simulink model "micromodelswil"  (R2021a)
settings: Solver=FixedStepAuto  StartTime=0.0  StopTime=inf  FixedStep=0.05  RelTol=1e-3
undefined symbols (not defined in the file): Angular, Linear
libraries: robotlib x21
settings Model: Creator=refulgent  LastModifiedBy=refulgent
settings OptimizationCC: EnhancedBackFolding=on  PassReuseOutputArgsAs=Individual arguments  ZeroExternalMemoryAtStartup=off  ZeroInternalMemoryAtStartup=off  MaxStackSize=64  OptimizeBlockOrder=speed  DifferentSizesBufferReuse=on  OptimizationCustomize=off  EfficientTunableParamExpr=on
settings DebuggingCC: ParameterTunabilityLossMsg=error
settings HardwareCC: ProdBitPerPointer=32  ProdBitPerSizeT=32  ProdBitPerPtrDiffT=32  ProdLargestAtomicFloat=None  ProdIntDivRoundTo=Undefined  ProdEndianess=Unspecified  ProdWordSize=32  ProdHWDeviceType=Generic->Unspecified (assume 32-bit Generic)
settings SFSimCC: MATLABDynamicMemAlloc=off
settings RTWCC: SystemTargetFile=ert.tlc  HardwareBoard=Robot Operating System (ROS)  TLCOptions="-aInlineSetEventsForThisBaseRateFcn=TLC_FALSE -aSuppressMultiTaskScheduler=TLC_FALSE  -aRateBasedStepFcn=0"  TemplateMakefile=ert_default_tmf  Toolchain=Catkin  TargetLang=C++
settings CodeAppCC: ForceParamTrailComments=on  IgnoreCustomStorageClasses=off  OperatorAnnotations=on  SimulinkDataObjDesc=on  SFDataObjDesc=on  InsertBlockDesc=on

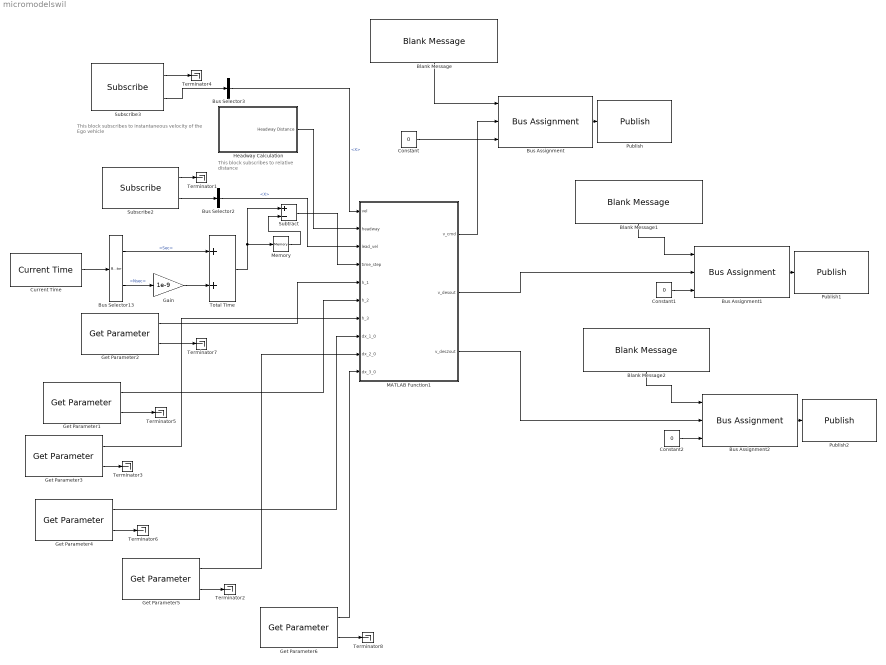
== system micromodelswil ==
  note: This block subscribes to
      | instantaneous velocity of the Ego vehicle
  note: This block subscribes
      | to relative distance
  Blank Message : robotlib/Blank Message  messageClass=Message  entityType=geometry_msgs/Twist  messageType=geometry_msgs/Twist  SampleTime=inf  legacyBusStruct=off
  Blank Message1 : robotlib/Blank Message  messageClass=Message  entityType=geometry_msgs/Twist  messageType=geometry_msgs/Twist  SampleTime=inf  legacyBusStruct=off
  Blank Message2 : robotlib/Blank Message  messageClass=Message  entityType=geometry_msgs/Twist  messageType=geometry_msgs/Twist  SampleTime=inf  legacyBusStruct=off
  Bus Assignment : BusAssignment  AssignedSignals=Linear.X,Angular.Z
  Bus Assignment1 : BusAssignment  AssignedSignals=Linear.X,Angular.Z
  Bus Assignment2 : BusAssignment  AssignedSignals=Linear.X,Angular.Z
  Bus Selector13 : BusSelector  OutputSignals=Sec,Nsec
  Bus Selector2 : BusSelector  OutputSignals=Linear.X
  Bus Selector3 : BusSelector  OutputSignals=Linear.X
  Constant : Constant  Value=0
  Constant1 : Constant  Value=0
  Constant2 : Constant  Value=0
  Current Time : robotlib/Current Time  OutputFormat=bus  SampleTime=-1  ModelName=micromodelswil
      settings: SourceProductBaseCode=RR
  Gain : Gain  Gain=1e-9
  Get Parameter1 : robotlib/Get Parameter  ParameterSource=Specify your own  ParameterName=th2  ParameterType=double  ParameterMaxArrayLength=16  ParameterInitialValue=1.2  SampleTime=-1  ShowErrorCodeOutput=on  ModelName=micromodelswil  BlockId=ParamGet_micromodelswil_55
      settings: SourceProductBaseCode=RR
  Get Parameter2 : robotlib/Get Parameter  ParameterSource=Specify your own  ParameterName=th1  ParameterType=double  ParameterMaxArrayLength=16  ParameterInitialValue=0.4  SampleTime=-1  ShowErrorCodeOutput=on  ModelName=micromodelswil  BlockId=ParamGet_micromodelswil_56
      settings: SourceProductBaseCode=RR
  Get Parameter3 : robotlib/Get Parameter  ParameterSource=Specify your own  ParameterName=th3  ParameterType=double  ParameterMaxArrayLength=16  ParameterInitialValue=1.8  SampleTime=-1  ShowErrorCodeOutput=on  ModelName=micromodelswil  BlockId=ParamGet_micromodelswil_57
      settings: SourceProductBaseCode=RR
  Get Parameter4 : robotlib/Get Parameter  ParameterSource=Specify your own  ParameterName=w1  ParameterType=double  ParameterMaxArrayLength=16  ParameterInitialValue=4.5  SampleTime=-1  ShowErrorCodeOutput=on  ModelName=micromodelswil  BlockId=ParamGet_micromodelswil_58
      settings: SourceProductBaseCode=RR
  Get Parameter5 : robotlib/Get Parameter  ParameterSource=Specify your own  ParameterName=w2  ParameterType=double  ParameterMaxArrayLength=16  ParameterInitialValue=5.25  SampleTime=-1  ShowErrorCodeOutput=on  ModelName=micromodelswil  BlockId=ParamGet_micromodelswil_73
      settings: SourceProductBaseCode=RR
  Get Parameter6 : robotlib/Get Parameter  ParameterSource=Specify your own  ParameterName=w3  ParameterType=double  ParameterMaxArrayLength=16  ParameterInitialValue=6.0  SampleTime=-1  ShowErrorCodeOutput=on  ModelName=micromodelswil  BlockId=ParamGet_micromodelswil_75
      settings: SourceProductBaseCode=RR
  Headway Calculation : Subsystem
  MATLAB Function1 : MATLAB Function  TreatAsAtomicUnit=on
  Memory : Memory
  Publish : robotlib/Publish  topicSource=Specify your own  topic=cmd_vel  messageType=geometry_msgs/Twist  legacyBusStruct=off  messageQueueLength=1
  Publish1 : robotlib/Publish  topicSource=Specify your own  topic=v_des  messageType=geometry_msgs/Twist  legacyBusStruct=off  messageQueueLength=1
  Publish2 : robotlib/Publish  topicSource=Specify your own  topic=v_des2  messageType=geometry_msgs/Twist  legacyBusStruct=off  messageQueueLength=1
  Subscribe2 : robotlib/Subscribe  topicSource=Specify your own  topic=leader_vel  messageType=geometry_msgs/Twist  SampleTime=-1  legacyBusStruct=off  messageQueueLength=1
  Subscribe3 : robotlib/Subscribe  topicSource=Specify your own  topic=vel  messageType=geometry_msgs/Twist  SampleTime=-1  legacyBusStruct=off  messageQueueLength=1
  Subtract : Sum  Inputs=+-
  Terminator{1..8} (8 alike) : Terminator
  Total Time : Sum
  wires:
  Bus Selector13/2 -> Gain/1  "<Nsec>"
  Bus Selector13/1 -> Total Time/1  "<Sec>"
  Gain/1 -> Total Time/2
  Current Time/1 -> Bus Selector13/1
  Total Time/1 -> Memory/1, Subtract/1
  Memory/1 -> Subtract/2
  Subtract/1 -> MATLAB Function1/4(time_step)
  Subscribe3/1 -> Terminator4/1
  Subscribe3/2 -> Bus Selector3/1
  Bus Selector3/1 -> MATLAB Function1/1(vel)  "<X>"
  Bus Assignment/1 -> Publish/1
  Constant/1 -> Bus Assignment/3
  MATLAB Function1/1(v_cmd) -> Bus Assignment/2
  Blank Message/1 -> Bus Assignment/1
  Subscribe2/1 -> Terminator1/1
  Bus Selector2/1 -> MATLAB Function1/3(lead_vel)  "<X>"
  Subscribe2/2 -> Bus Selector2/1
  Headway Calculation/1(Headway Distance) -> MATLAB Function1/2(headway)
  Get Parameter3/2 -> Terminator3/1
  Get Parameter1/1 -> MATLAB Function1/6(h_2)
  Get Parameter3/1 -> MATLAB Function1/7(h_3)
  Get Parameter1/2 -> Terminator5/1
  Get Parameter2/1 -> MATLAB Function1/5(h_1)
  Get Parameter4/2 -> Terminator6/1
  Get Parameter2/2 -> Terminator7/1
  Get Parameter4/1 -> MATLAB Function1/8(dx_1_0)
  Blank Message1/1 -> Bus Assignment1/1
  MATLAB Function1/2(v_desout) -> Bus Assignment1/2
  Constant1/1 -> Bus Assignment1/3
  Bus Assignment1/1 -> Publish1/1
  Bus Assignment2/1 -> Publish2/1
  Constant2/1 -> Bus Assignment2/3
  MATLAB Function1/3(v_des2out) -> Bus Assignment2/2
  Blank Message2/1 -> Bus Assignment2/1
  Get Parameter5/1 -> MATLAB Function1/9(dx_2_0)
  Get Parameter5/2 -> Terminator2/1
  Get Parameter6/2 -> Terminator8/1
  Get Parameter6/1 -> MATLAB Function1/10(dx_3_0)

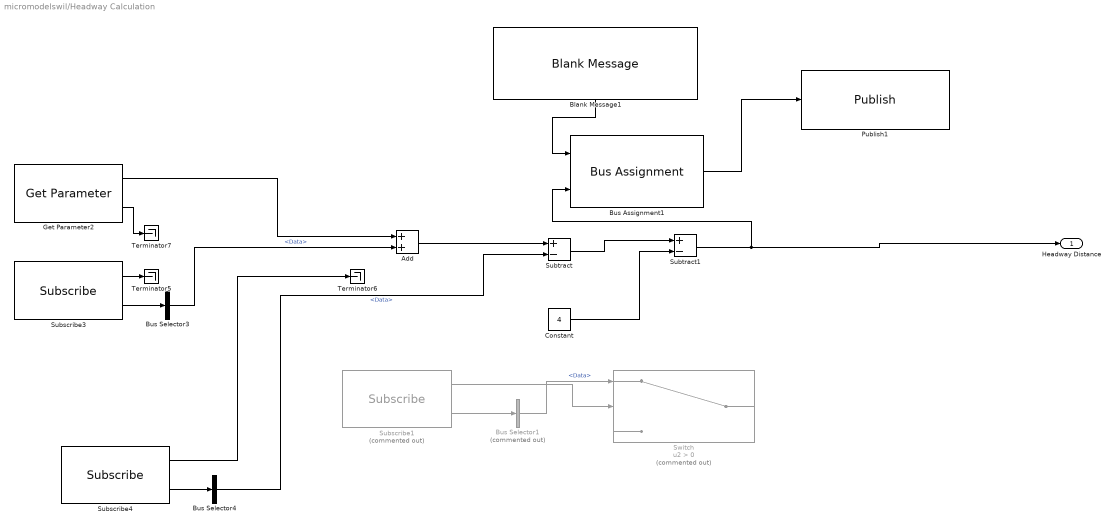
== system micromodelswil/Headway Calculation ==
  Add : Sum
  Blank Message1 : robotlib/Blank Message  messageClass=Message  entityType=std_msgs/Float64  messageType=std_msgs/Float64  SampleTime=inf  legacyBusStruct=off
  Bus Assignment1 : BusAssignment  AssignedSignals=Data
  Bus Selector1 : BusSelector  Commented=on  OutputSignals=Data
  Bus Selector3 : BusSelector  OutputSignals=Data
  Bus Selector4 : BusSelector  OutputSignals=Data
  Constant : Constant  Value=4
  Get Parameter2 : robotlib/Get Parameter  ParameterSource=Specify your own  ParameterName=init_gap  ParameterType=double  ParameterMaxArrayLength=16  ParameterInitialValue=30.0  SampleTime=-1  ShowErrorCodeOutput=on  ModelName=micromodelswil  BlockId=ParamGet_micromodelswil_39
      settings: SourceProductBaseCode=RR
  Publish1 : robotlib/Publish  topicSource=Specify your own  topic=headway_est  messageType=std_msgs/Float64  legacyBusStruct=off  messageQueueLength=1
  Subscribe1 : robotlib/Subscribe  Commented=on  topicSource=Specify your own  topic=headway  messageType=std_msgs/Float64  SampleTime=-1  legacyBusStruct=off  messageQueueLength=1
  Subscribe3 : robotlib/Subscribe  topicSource=Specify your own  topic=leader_dist_x  messageType=std_msgs/Float64  SampleTime=-1  legacyBusStruct=off  messageQueueLength=1
  Subscribe4 : robotlib/Subscribe  topicSource=Specify your own  topic=dist_x  messageType=std_msgs/Float64  SampleTime=-1  legacyBusStruct=off  messageQueueLength=1
  Subtract : Sum  Inputs=+-
  Subtract1 : Sum  Inputs=+-
  Switch : Switch  Commented=on  Criteria=u2 > Threshold
  Terminator5 : Terminator
  Terminator6 : Terminator
  Terminator7 : Terminator
  Headway Distance : Outport
  wires:
  Bus Selector3/1 -> Add/2  "<Data>"
  Subscribe1/2 -> Bus Selector1/1
  Subscribe3/2 -> Bus Selector3/1
  Subscribe4/1 -> Terminator6/1
  Bus Selector1/1 -> Switch/1  "<Data>"
  Subscribe1/1 -> Switch/2
  Bus Selector4/1 -> Subtract/2  "<Data>"
  Get Parameter2/2 -> Terminator7/1
  Subscribe4/2 -> Bus Selector4/1
  Get Parameter2/1 -> Add/1
  Subscribe3/1 -> Terminator5/1
  Add/1 -> Subtract/1
  Subtract/1 -> Subtract1/1
  Blank Message1/1 -> Bus Assignment1/1
  Bus Assignment1/1 -> Publish1/1
  Subtract1/1 -> Bus Assignment1/2, Headway Distance/1
  Constant/1 -> Subtract1/2

== matlab function micromodelswil/MATLAB Function1 ==
  data: vel input; v_cmd output; v_desout output; headway input; lead_vel input; time_step input; h_1 input; h_2 input; h_3 input; dx_1_0 input; v_des2out output; dx_2_0 input; dx_3_0 input
function [v_cmd, v_desout, v_des2out]  = Micromodel(vel, headway, lead_vel, time_step, h_1, h_2, h_3, dx_1_0, dx_2_0, dx_3_0)
%% Compute the desired acceleration by the Micromodel controller.
% This model requires memory from previous time steps to properly function.
% To achieve this, we pass the variables to be stored in memory as inputs
% to the function, and return the updated values as outputs from it. These
% parameters should be initialized as follows:
% >>> d1 = 1;
% >>> d2 = 1;
% >>> v_des2 = -1;
% >>> time_avg_target = [];
% If you would like to convert this model from an acceleration controller
% to a velocity controller, simply replace "acceleration" in the above
% function definition with "v_cmd".
% Parameters
% ----------
% vel : float
%     the speed of the ego vehicle
% headway : float
%     bumper-to-bumper gap
% lead_vel : float
%     speed of vehicle in front
% time_step : float
%     the average time (in seconds) in between consecutive updates
% d1 : {0, 1}
%     specifies whether the vehicle is in or out of the too fast zone at 
%     the previous time. Initialized as 1.
% d2 : {0, 1}
%     specifies whether the vehicle already adjusted speed or not.
%     Initialized as 1.
% v_des2 : float
%     local target speed. Initialize at -1.
% time_avg_target : list of float
%     a buffer of leader speeds at previous time steps
% Returns
% -------
% (float, float, float, float, list of float)
%     the desired acceleration and updated d1, d2, v_des2, and 
%     time_avg_target terms
%% model parameters
max_accel = 1.5; max_deaccel = -3;
v_fast = 40;
% to be optimized
%period = 65; 
params_1 = 2; params_3 = 5; params_3_1 = 1.3; params_1_1 = 1.1;
reduction = 0.8;
increase = 0.01;
%% Follower Stopper parameters
% h_1 = 0.4;
% h_2 = 1.2;
% h_3 = 1.8;
% dx_1_0 = 4.5;
%dx_2_0 = 5.25;
%dx_3_0 = 6.0;
d_1 = 1.5;
d_2 = 1.0;
d_3 = 0.5;
%% Persistent variables
persistent v_des2
persistent d1
persistent d2
persistent time_avg_target
persistent t_length
if isempty(time_avg_target)
    t_length= 1;
    time_avg_target = zeros(1, 1280);% Data Rate = 20 Hz, To consider 64 seconds, 20*64 data points are required
    time_avg_target(1280)= lead_vel;
    d1 = 1;
    d2 = 1;
else
    time_avg_target = [time_avg_target(2:end),lead_vel];
    if(t_length < 1280)
        t_length= t_length + 1;
    end
end
%% Choose the desired speed based on the Follower Stopper model.
% Create reference values for global target speed.
% time_avg_target(end+1) = lead_vel
v_des = sum(time_avg_target)/t_length;
v_des2 = v_des;
% % Create local target speed.
% if v_des2 == -1
%     v_des2 = v_des;
% end
if (d1 == 0) && (d2 == 0)
    v_des2 = min(v_des2 * reduction, v_des * reduction);
    d2 = 1;
else
    v_des2 = min(v_des2 * (1 + increase * time_step), v_des);
end
% Add a filter for free flow.
if lead_vel > 20
    v_des2 = lead_vel;
elseif lead_vel > 15
    v_des2 = v_des2 + (lead_vel - v_des2) * (lead_vel - 15) / 5;
end
% Compute the hysteresis and the wrapper.
dx = headway;
dv_minus = min(lead_vel - vel, 0);
v = min(max(lead_vel, 0), v_des);
dx_1 = 1 / (2 * d_1) * dv_minus ^ 2 + max(dx_1_0, h_1 * vel);
dx_2 = 1 / (2 * d_2) * dv_minus ^ 2 + max(dx_2_0, h_2 * vel);
dx_3 = 1 / (2 * d_3) * dv_minus ^ 2 + max(dx_3_0, h_3 * vel);
dx_5 = max(dx_3_0 * params_3, params_3_1 * dx_3);
dx_4 = max(dx_3_0 * params_1, params_1_1 * dx_3);
if dx >= dx_5
    v_cmd = min(v_des * (1 + (dx - dx_5) / (dx_5)), v_fast);
elseif dx >= dx_4
    v_cmd = v_des + min(0, (v_des2 - v_des) * (dx_5 - dx) / (dx_5 - dx_4));
elseif dx >= dx_3
    v_cmd = v_des2;
elseif dx >= dx_2
    v_cmd = v + (v_des2 - v) * (dx - dx_2) / (dx_3 - dx_2);
elseif dx >= dx_1
    v_cmd = v * (dx - dx_1) / (dx_2 - dx_1);
    d1 = 1;
    d2 = 0;
else
    v_cmd = 0;
    d1 = 0;
end
%% Convert speed to acceleration.
acceleration = (v_cmd - vel) / time_step;
acceleration = min(max(acceleration, -abs(max_deaccel)), max_accel);
v_desout = v_des;
v_des2out = v_des2;
end
